simulink subsystem "HallSensor"  (R2023a)
settings: Solver=VariableStepAuto  StartTime=0.0  StopTime=10.0  RelTol=1e-3
model mask{speed_coef=0.2, angle_coef=2}
  mask prompts: speed_coef "Speed_coeff"; angle_coef "Angle_coeff"
undefined symbols (not defined in the file): KspeedSens
settings Model: Creator=User  LastModifiedBy=User

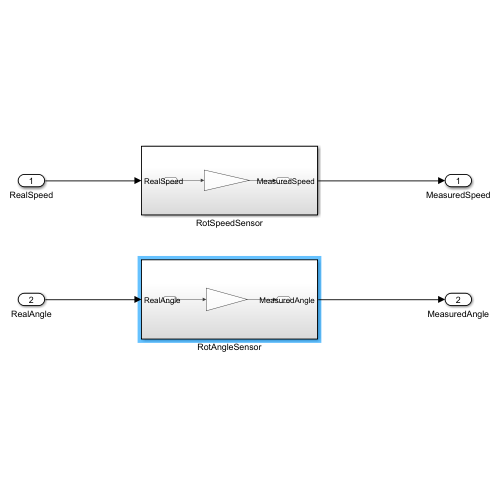
[thumbnail: Simulink's stored preview of the top-level diagram]
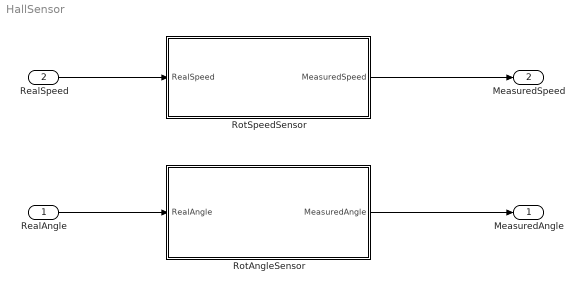
== system HallSensor ==
  RealAngle : Inport
  RealSpeed : Inport  Port=2
  RotAngleSensor : Subsystem
  RotSpeedSensor : Subsystem
  MeasuredAngle : Outport
  MeasuredSpeed : Outport  Port=2
  wires:
  RealSpeed/1 -> RotSpeedSensor/1(RealSpeed)
  RotSpeedSensor/1(MeasuredSpeed) -> MeasuredSpeed/1
  RotAngleSensor/1(MeasuredAngle) -> MeasuredAngle/1
  RealAngle/1 -> RotAngleSensor/1(RealAngle)

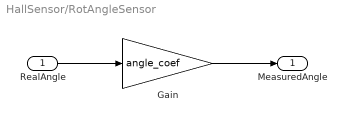
== system HallSensor/RotAngleSensor ==
  RealAngle : Inport
  Gain : Gain  Gain=angle_coef
  MeasuredAngle : Outport
  wires:
  RealAngle/1 -> Gain/1
  Gain/1 -> MeasuredAngle/1

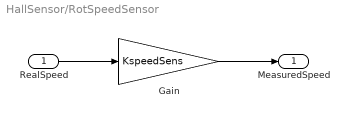
== system HallSensor/RotSpeedSensor ==
  RealSpeed : Inport
  Gain : Gain  Gain=KspeedSens
  MeasuredSpeed : Outport
  wires:
  RealSpeed/1 -> Gain/1
  Gain/1 -> MeasuredSpeed/1
